simulink model "motorsimu"  (R2022b)
settings: Solver=VariableStepAuto  StartTime=0.0  StopTime=10.0  RelTol=1e-3
undefined symbols (not defined in the file or in its folder): A, d, n
settings Model: Creator=Fatih  LastModifiedBy=Fatih

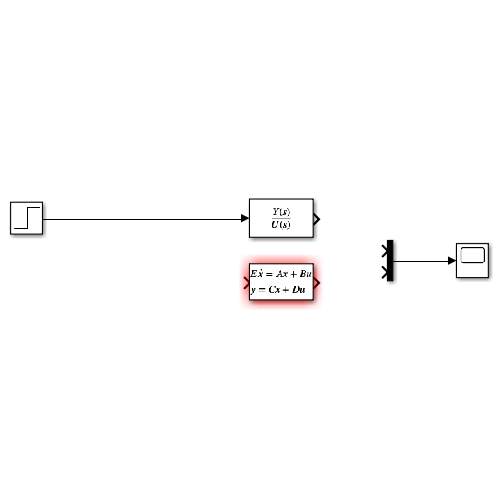
[thumbnail: Simulink's stored preview of the top-level diagram]
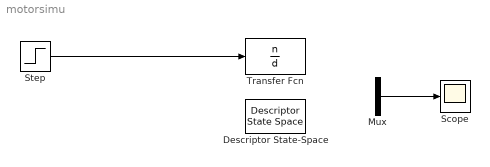
== system motorsimu ==
  Descriptor State-Space : DescriptorStateSpace  A=A
  Mux : Mux  Inputs=2
  Scope : Scope
  Step : Step  SampleTime=0
  Transfer Fcn : TransferFcn  Numerator=n  Denominator=d
  wires:
  Step/1 -> Transfer Fcn/1
  Mux/1 -> Scope/1
